simulink model "msd_sfun_model_sf_control"  (R2015a)
settings: Solver=ode45  StartTime=0.0  StopTime=35  RelTol=1e-3
settings Model: Creator=Arnab Banerjee  LastModifiedBy=Arnab Banerjee

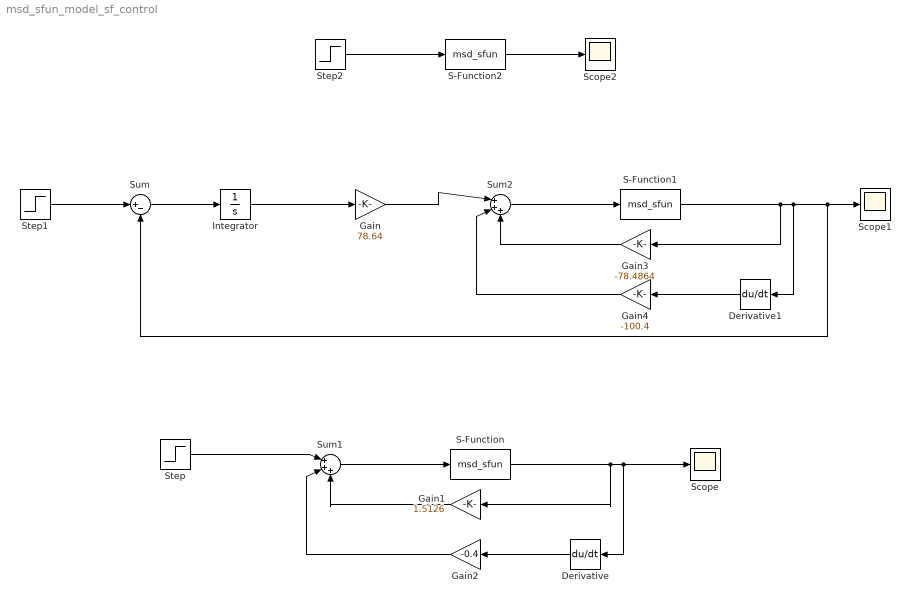
== system msd_sfun_model_sf_control ==
  Derivative : Derivative
  Derivative1 : Derivative
  Gain : Gain  Gain=78.64
  Gain1 : Gain  Gain=1.5126
  Gain2 : Gain  Gain=-0.4
  Gain3 : Gain  Gain=-78.4864
  Gain4 : Gain  Gain=-100.4
  Integrator : Integrator
  S-Function : S-Function  FunctionName=msd_sfun
  S-Function1 : S-Function  FunctionName=msd_sfun
  S-Function2 : S-Function  FunctionName=msd_sfun
  Scope : Scope
  Scope1 : Scope
      settings: YMin=0.112357  YMax=0.1124
  Scope2 : Scope
      settings: SaveName=ScopeData2
  Step : Step  Time=0  SampleTime=0
  Step1 : Step  Time=0  SampleTime=0
  Step2 : Step  Time=0  SampleTime=0
  Sum : Sum  Inputs=|+-
  Sum1 : Sum  Inputs=|+++
  Sum2 : Sum  Inputs=|+++
  wires:
  S-Function/1 -> Gain1/1, Derivative/1, Scope/1
  Sum1/1 -> S-Function/1
  Gain1/1 -> Sum1/3
  Gain2/1 -> Sum1/2
  Derivative/1 -> Gain2/1
  Step/1 -> Sum1/1
  Integrator/1 -> Gain/1
  Step1/1 -> Sum/1
  Sum/1 -> Integrator/1
  S-Function1/1 -> Gain3/1, Derivative1/1, Sum/2, Scope1/1
  Sum2/1 -> S-Function1/1
  Gain3/1 -> Sum2/3
  Gain4/1 -> Sum2/2
  Derivative1/1 -> Gain4/1
  Gain/1 -> Sum2/1
  Step2/1 -> S-Function2/1
  S-Function2/1 -> Scope2/1
